simulink model "gbyk_rwd_tgtprob"  (R2015a)
settings: Solver=ode4  SolverMode=MultiTasking  StartTime=0.0  StopTime=inf  FixedStep=BKIN_STEP_TIME  RelTol=1e-3
StartFcn:
  |  warndlg('Dexterit-E models cannot run under simulation. Please compile your model and run it from within Dexterit-E.');set_param(bdroot,'SimulationCommand','stop')
model workspace (MAT data in the model file):
  BKIN_STEP_TIME = 0.00025
  col_x = 1
  col_y = 2
  INIT_COLOR = 5
  DELAY_POST_TRIAL = 8
  BKIN_KINEMATIC_FRAME_SIZE = 400
  HIT_COLOR = 6
  E_NO_EVENT = 0
  START_TARGET_COL = 1
  TARGET1_COL = 2
  TARGET2_COL = 3
  RWD_TARGET1_COL = 4
  RWD_TARGET2_COL = 5
  MAX_REACH_TIME_COL = 7
  K_DELAY_FIXED = 3
  K_DELAY_RAND = 4
  K_TRIGGER_VEL = 5
  K_TRIGGER_POS = 6
  K_THRESH_VELMAX = 7
  E_NEW_TRIAL = 1
  E_STAY_START = 2
  E_TARGET_TRIGGER = 5
  E_HIT_TARGET = 10
  E_MISS_TARGET = 11
  K_REWARD_VAL = 1
  VISUAL_RADIUS = 3
  LOGICAL_RADIUS = 4
  STROKE_WIDTH = 7
  TEXT_COLOR = 8
  LABEL_HEIGHT = 10
  E_TOO_SLOW = 20
  K_TONE_HIT_FREQUENCY = 8
  K_TONE_HIT_DURATION = 9
  K_TONE_ERROR_FREQUENCY = 12
  K_TONE_ERROR_DURATION = 13
  K_SCORETEXT_ROW = 2
  LABEL = 9
  E_TARGETS_ON = 3
  K_TONE_GO_FREQUENCY = 10
  K_TONE_GO_DURATION = 11
  DISPLAY_TRIAL_COL = 9
  E_SHOW_INSTRUCT = 25
  E_SHOW_SCORE = 26
  INSTRUCT_PAUSE_BTN = 2
  TARGET1_PROB_COL = 6
  TARGET_SIZE = 11
libraries: Video x6, slrtlib x5, General x3, KINARM_general x3, simulink x1, xpcnilib x1
CloseFcn:
  | rtwprivate ssgencode ModelCloseRequest b2lab2d
settings Model: ModifiedComment=chris -- Wed Feb 16 09:18:30 2005 -- Version 1.1384  ModifiedHistory=Feb 16/05 - Add error repeat, add offset ramp  ExtModeArmWhenConnect=off  ExtModeLogAll=off  Creator=Chris Grebeldinger  LastModifiedBy=User
settings SolverCC: EnableConcurrentExecution=on  AutoInsertRateTranBlk=on
settings DataIOCC: LimitDataPoints=off  SignalLoggingSaveFormat=ModelDataLogs  SaveOutput=off  SaveTime=off  SignalLoggingName=sigsOut
settings OptimizationCC: BlockReduction=off  BooleanDataType=off  OptimizeBlockIOStorage=off  BufferReuse=off  GlobalBufferReuse=off  ExpressionFolding=off  ExpressionDepthLimit=2147483647  LocalBlockOutputs=off  InitFltsAndDblsToZero=on
settings DebuggingCC: SaveWithParameterizedLinksMsg=none  UnderspecifiedInitializationDetection=Classic  MergeDetectMultiDrivingBlocksExec=none  SignalResolutionControl=TryResolveAllWithWarning  MultiTaskDSMMsg=warning  FcnCallInpInsideContextMsg=UseLocalSettings  StateNameClashWarn=warning  StrictBusMsg=ErrorOnBusTreatedAsVector
settings HardwareCC: ProdIntDivRoundTo=Zero  ProdEndianess=LittleEndian  ProdLongLongMode=on  ProdHWDeviceType=Generic->32-bit x86 compatible  TargetHWDeviceType=32-bit Generic
settings SFSimCC: SimCustomHeaderCode="#include \"stdlib.h\""  SFSimEcho=off  SimParseCustomCode=off
settings RTWCC: SystemTargetFile=slrt.tlc  TemplateMakefile=slrt_default_tmf  Description=Simulink Real-Time  CustomSourceCode="#include \"stdlib.h\""  RTWCompilerOptimization=on
settings CodeAppCC: MaxIdLength=63
settings SimulinkRealTimeCC: TargetFcnLib=ansi_tfl_tmw.mat  GeneratePreprocessorConditionals=Disable all  xPCisDownloadable=off  xPCisDefaultEnv=off

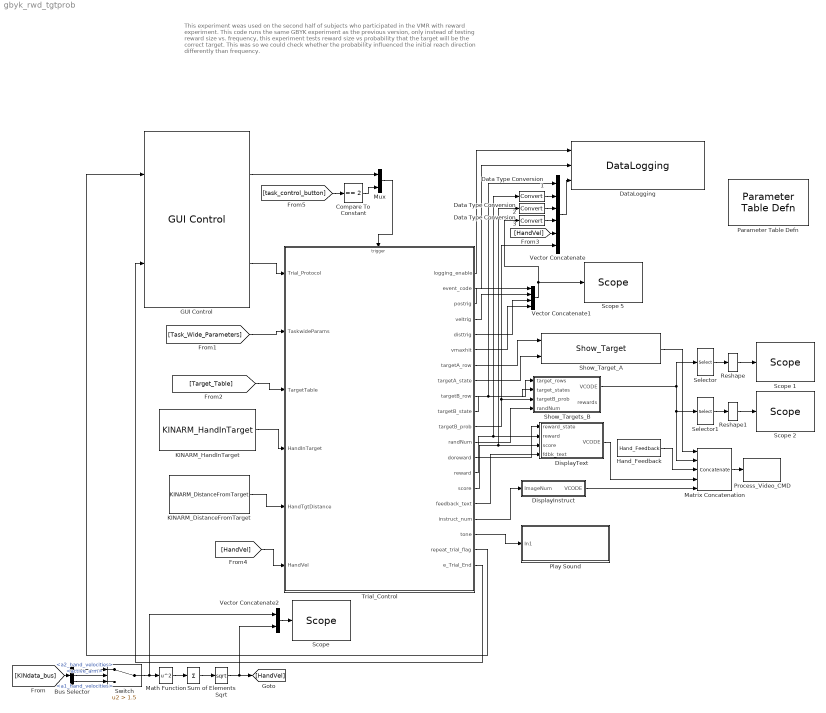
== system gbyk_rwd_tgtprob ==
  note: This experiment weas used on the second half of subjects who participated in the
      | VMR with reward experiment. This code runs the same GBYK experiment as the
      | previous version, only instead of testing reward size vs. frequency, this experiment
      | tests reward size vs probability that the target will be the correct target. This was
      | so we could check whether the probability influenced the initial reach direction
      | differently than frequency.
  Bus Selector : BusSelector  OutputSignals=Robot2.a2_hand_velocities,KINDataGeneral.active_arm,Robot1.a1_hand_velocities
  Compare To Constant : simulink/Logic and Bit Operations/Compare To Constant  relop===  const=2  OutDataTypeStr=boolean
  Data Type Conversion1 : DataTypeConversion
  Data Type Conversion2 : DataTypeConversion
  Data Type Conversion3 : DataTypeConversion
  DataLogging : General/DataLogging  log_event_codes=on  log_analog_inputs=on  show_time_remaining=off
      link override Poll KINARM/EPTorqueCMD: GotoTag=KINARMEPTorqueCMD
      link override Poll KINARM/TorqueCMD: GotoTag=KINARMTorqueCMD
  DisplayInstruct : Subsystem
  DisplayText : Subsystem
  GUI Control : General/GUI Control  target_type_str=Circle  Target_Type=1  XYcols=[1 2]  Vcols=3  Lcols=4  indices_padding=[0 0 0 0;0 0 0 0]  task_version=1.0  show_repeat_trial_flag=on  target_table_rows=32  load_table_rows=20  tp_table_rows=100
  Hand_Feedback : KINARM_general/Hand_Feedback  feedback_cntl_src=none
  KINARM_DistanceFromTarget : KINARM_general/KINARM_DistanceFromTarget  use_dominant_hand=on
  KINARM_HandInTarget : KINARM_general/KINARM_HandInTarget  use_dominant_hand=on  target_type=Circle  num_states=1  attribcol1=[LOGICAL_RADIUS]  attribcol2=[4]  attribcol3=[5]  attribcol4=[6]  attribcol5=[0]
  Math Function : Math  Operator=square  SaturateOnIntegerOverflow=on
  Matrix Concatenation : Concatenate  NumInputs=5  Mode=Multidimensional array
  Mux : Mux  Inputs=2
  Parameter Table Defn : General/Parameter Table Defn  ShowInLibBrowser=0
  Play Sound : Subsystem
  Process_Video_CMD : Video/Process_Video_CMD  video_delay=50
  Reshape : Reshape
  Reshape1 : Reshape
  "Scope " : slrtlib/Displays and Logging/Scope   scopeno=1  scopetype=Target  autostart=on  viewmode=Numerical  formatstr='%15.6f'  grid=on  ylimits=[0,0]  nosamples=250  noprepostsamples=0  interleave=1  triggermode=FreeRun  triggersignal=1  trigsignalfromport=off  triggerlevel=0.0  triggerslope=Either  triggerscope=1  triggersample=0  filename=data.dat  mode=Lazy  writesize=512  autorestart=off  dynamicfilemode=off  maxwritefilesize=512*1024^2
  Scope 1 : slrtlib/Displays and Logging/Scope   scopeno=2  scopetype=Target  autostart=on  viewmode=Numerical  formatstr='%15.6f'  grid=on  ylimits=[0,0]  nosamples=250  noprepostsamples=0  interleave=1  triggermode=FreeRun  triggersignal=1  trigsignalfromport=off  triggerlevel=0.0  triggerslope=Either  triggerscope=1  triggersample=0  filename=data.dat  mode=Lazy  writesize=512  autorestart=off  dynamicfilemode=off  maxwritefilesize=512*1024^2
  Scope 2 : slrtlib/Displays and Logging/Scope   scopeno=3  scopetype=Target  autostart=on  viewmode=Numerical  formatstr='%15.6f'  grid=on  ylimits=[0,0]  nosamples=250  noprepostsamples=0  interleave=1  triggermode=FreeRun  triggersignal=1  trigsignalfromport=off  triggerlevel=0.0  triggerslope=Either  triggerscope=1  triggersample=0  filename=data.dat  mode=Lazy  writesize=512  autorestart=off  dynamicfilemode=off  maxwritefilesize=512*1024^2
  Scope 5 : slrtlib/Displays and Logging/Scope   scopeno=6  scopetype=Target  autostart=on  viewmode=Numerical  formatstr='%15.6f'  grid=on  ylimits=[0,0]  nosamples=250  noprepostsamples=0  interleave=1  triggermode=FreeRun  triggersignal=1  trigsignalfromport=off  triggerlevel=0.0  triggerslope=Either  triggerscope=1  triggersample=0  filename=data.dat  mode=Lazy  writesize=512  autorestart=off  dynamicfilemode=off  maxwritefilesize=512*1024^2
  Selector : Selector  NumberOfDimensions=2  InputPortWidth=3  IndexOptions=Index vector (dialog),Index vector (dialog)  Indices=[1:2],[2 3 4 15 16]  OutputSizes=1,1
  Selector1 : Selector  NumberOfDimensions=2  InputPortWidth=3  IndexOptions=Index vector (dialog),Index vector (dialog)  Indices=[3:4],[2 3 4 9]  OutputSizes=1,1
  Show_Target_A : Video/Show_Target  target_type=Circle  num_states=2  attribcol1=[INIT_COLOR 0 0 VISUAL_RADIUS]  attribcol2=[HIT_COLOR 0 0 VISUAL_RADIUS]  attribcol3=[0 0 0 0]  attribcol4=[0 0 0 0]  attribcol5=[0 0 24 0]  stateindices_padding=[0 0 0 0 0 0 0;0 0 0 0 0 0 0;0 0 0 0 0 0 0;0 0 0 0 0 0 0;0 0 0 0 0 0 0]  source=dialog  opacity=100  target_display=Both subject and operator displays  num_col=4
  Show_Targets_B : Subsystem
  Sqrt : Sqrt  SaturateOnIntegerOverflow=on
  Sum of Elements : Sum  Inputs=+
  Switch : Switch  Criteria=u2 > Threshold  Threshold=1.5
  Trial_Control : Stateflow chart  TreatAsAtomicUnit=on
  Vector Concatenate : Concatenate  NumInputs=6
  Vector Concatenate1 : Concatenate  NumInputs=4
  Vector Concatenate2 : Concatenate
  wires:
  KINARM_HandInTarget/1 -> Trial_Control/4(HandInTarget)
  Show_Target_A/1 -> Matrix Concatenation/1
  GUI Control/2 -> Trial_Control/1(Trial_Protocol)
  Trial_Control/19(repeat_trial_flag) -> GUI Control/1
  Trial_Control/8(targetA_state) -> Show_Target_A/2
  Trial_Control/7(targetA_row) -> Show_Target_A/1
  Matrix Concatenation/1 -> Process_Video_CMD/1
  Hand_Feedback/1 -> Matrix Concatenation/3
  Show_Targets_B/1(VCODE) -> Selector/1, Selector1/1, Matrix Concatenation/2
  Trial_Control/9(targetB_row) -> Show_Targets_B/1(target_rows)
  Trial_Control/10(targetB_state) -> Vector Concatenate/1, Show_Targets_B/2(target_states)
  Trial_Control/1(logging_enable) -> DataLogging/1
  Trial_Control/2(event_code) -> DataLogging/2
  [KINdata_bus] -> Bus Selector/1
  KINARM_DistanceFromTarget/1 -> Trial_Control/5(HandTgtDistance)
  [Task_Wide_Parameters] -> Trial_Control/2(TaskwideParams)
  [Target_Table] -> Trial_Control/3(TargetTable)
  Trial_Control/13(doreward) -> DisplayText/1(reward_state)
  Trial_Control/20(e_Trial_End) -> GUI Control/2
  Trial_Control/14(reward) -> Data Type Conversion1/1, DisplayText/2(reward)
  Trial_Control/15(score) -> Data Type Conversion2/1, DisplayText/3(score)
  DisplayText/1(VCODE) -> Matrix Concatenation/4
  Vector Concatenate/1 -> DataLogging/3
  Data Type Conversion1/1 -> Vector Concatenate/2
  Data Type Conversion2/1 -> Vector Concatenate/3
  Trial_Control/16(feedback_text) -> DisplayText/4(fdbk_text)
  Selector/1 -> Reshape/1
  Reshape/1 -> Scope 1/1
  Trial_Control/3(postrig) -> Vector Concatenate1/1
  Trial_Control/4(veltrig) -> Vector Concatenate1/2
  Trial_Control/5(disttrig) -> Vector Concatenate1/3
  Trial_Control/6(vmaxhit) -> Vector Concatenate1/4
  Vector Concatenate1/1 -> Data Type Conversion3/1, Scope 5/1
  Data Type Conversion3/1 -> Vector Concatenate/4
  Vector Concatenate2/1 -> "Scope "/1
  Switch/1 -> Vector Concatenate2/1, Math Function/1
  Bus Selector/2 -> Switch/2  "<active_arm>"
  Bus Selector/3 -> Switch/3  "<a1_hand_velocities>"
  Bus Selector/1 -> Switch/1  "<a2_hand_velocities>"
  Math Function/1 -> Sum of Elements/1
  Sum of Elements/1 -> Sqrt/1
  [HandVel] -> Vector Concatenate/5
  [HandVel] -> Trial_Control/6(HandVel)
  Sqrt/1 -> Vector Concatenate2/2, [HandVel]
  Trial_Control/17(instruct_num) -> DisplayInstruct/1(ImageNum)
  DisplayInstruct/1(VCODE) -> Matrix Concatenation/5
  GUI Control/1 -> Mux/1
  [task_control_button] -> Compare To Constant/1
  Compare To Constant/1 -> Mux/2
  Mux/1 -> Trial_Control/Trigger
  Trial_Control/11(targetB_prob) -> Vector Concatenate/6, Show_Targets_B/3(targetB_prob)
  Selector1/1 -> Reshape1/1
  Reshape1/1 -> Scope 2/1
  Trial_Control/12(randNum) -> Show_Targets_B/4(randNum)
  Trial_Control/18(tone) -> Play Sound/1(In1)

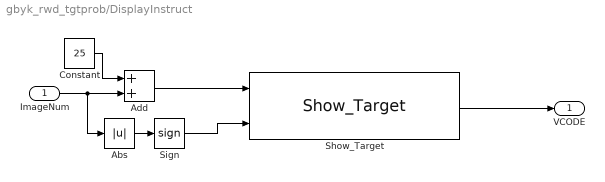
== system gbyk_rwd_tgtprob/DisplayInstruct ==
  ImageNum : Inport
  Abs : Abs
  Add : Sum
  Constant : Constant  Value=25
  Show_Target : Video/Show_Target  target_type=Rectangle  num_states=1  attribcol1=[INIT_COLOR 0 0 VISUAL_RADIUS LABEL_HEIGHT 0]  attribcol2=[6 6 0 3 0 0]  attribcol3=[0 0 0 0 0 0]  attribcol4=[0 0 0 0 0 0]  attribcol5=[0 0 24 0 0 0]  stateindices_padding=[0 0 0 0 0;0 0 0 0 0;0 0 0 0 0;0 0 0 0 0;0 0 0 0 0]  source=dialog  opacity=100  target_display=Both subject and operator displays  num_col=6
  Sign : Signum
  VCODE : Outport
  wires:
  ImageNum/1 -> Add/2, Abs/1
  Abs/1 -> Sign/1
  Show_Target/1 -> VCODE/1
  Add/1 -> Show_Target/1
  Constant/1 -> Add/1
  Sign/1 -> Show_Target/2

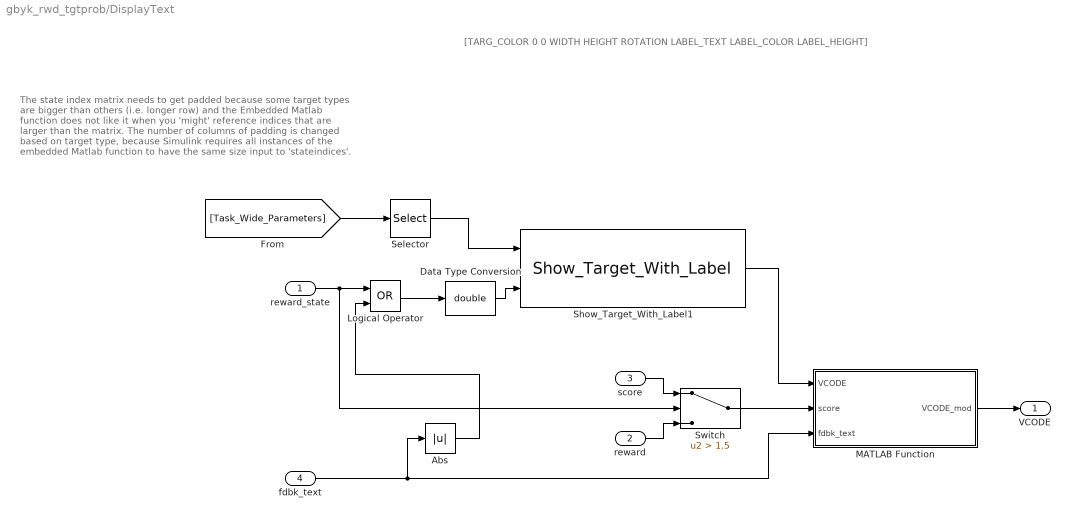
== system gbyk_rwd_tgtprob/DisplayText ==
  note: [TARG_COLOR 0 0 WIDTH HEIGHT ROTATION LABEL_TEXT LABEL_COLOR LABEL_HEIGHT]
  note: The state index matrix needs to get padded because
      | some target types are bigger than others (i.e. longer row)
      | and the Embedded Matlab function does not like it when you
      |  'might' reference indices that are larger than the matrix.
      |
      | The number of columns of padding is changed based on target
      | type, because Simulink requires all instances of the embedded
      | Matlab function to have the same size input to 'stateindices'.
  reward_state : Inport  OutDataTypeStr=double
  reward : Inport  Port=2  OutDataTypeStr=int32
  score : Inport  Port=3  OutDataTypeStr=int32
  fdbk_text : Inport  Port=4  OutDataTypeStr=int32
  Abs : Abs
  Data Type Conversion : DataTypeConversion  OutDataTypeStr=double
  Logical Operator : Logic  Operator=OR  AllPortsSameDT=off  OutDataTypeStr=boolean
  MATLAB Function : MATLAB Function  TreatAsAtomicUnit=on
  Selector : Selector  InputPortWidth=50  Indices=[K_SCORETEXT_ROW]
  Show_Target_With_Label1 : Video/Show_Target_With_Label  target_type=Rectangle  num_states=1  attribcol1=[INIT_COLOR 0 0 VISUAL_RADIUS VISUAL_RADIUS 0 LABEL TEXT_COLOR LABEL_HEIGHT]  attribcol2=[6 6 0 3 0 0 0 0 0]  attribcol3=[0 0 0 0 0 0 0 0 0]  attribcol4=[0 0 0 0 0 0 0 0 0]  attribcol5=[0 0 24 0 0 0 0 0 0]  stateindices_padding=[0 0;0 0;0 0;0 0;0 0]  source=dialog  opacity=100  target_display=Both subject and operator displays
  Switch : Switch  Criteria=u2 > Threshold  Threshold=1.5
  VCODE : Outport
  wires:
  reward_state/1 -> Logical Operator/1, Switch/2
  Show_Target_With_Label1/1 -> MATLAB Function/1(VCODE)
  MATLAB Function/1(VCODE_mod) -> VCODE/1
  score/1 -> Switch/1
  reward/1 -> Switch/3
  Switch/1 -> MATLAB Function/2(score)
  [Task_Wide_Parameters] -> Selector/1
  Selector/1 -> Show_Target_With_Label1/1
  Abs/1 -> Logical Operator/2
  Logical Operator/1 -> Data Type Conversion/1
  Data Type Conversion/1 -> Show_Target_With_Label1/2
  fdbk_text/1 -> MATLAB Function/3(fdbk_text), Abs/1

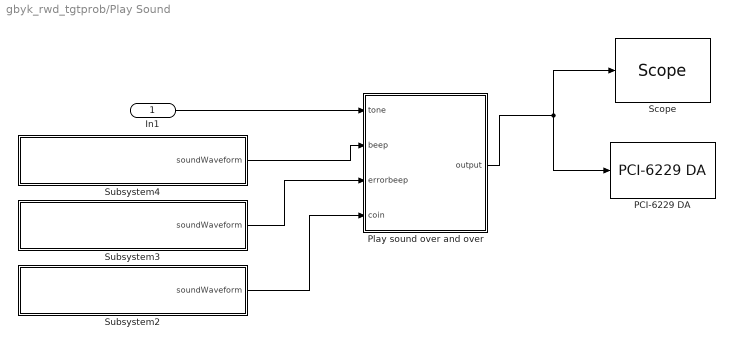
== system gbyk_rwd_tgtprob/Play Sound ==
  In1 : Inport
  PCI-6229 DA : xpcnilib/D//A/M Series/PCI-6229 DA  channel=[1]  reset=[1]  initValue=[0]  sampletime=-1  slot=-1
  Play sound over and over : MATLAB Function  TreatAsAtomicUnit=on
  "Scope " : slrtlib/Displays and Logging/Scope   scopeno=4  scopetype=Target  autostart=on  viewmode=Graphical redraw  formatstr='%15.6f'  grid=on  ylimits=[0,0]  nosamples=4000  noprepostsamples=0  interleave=1  triggermode=FreeRun  triggersignal=1  trigsignalfromport=off  triggerlevel=0.0  triggerslope=Either  triggerscope=1  triggersample=0  filename=data.dat  mode=Lazy  writesize=512  autorestart=off  dynamicfilemode=off  maxwritefilesize=512*1024^2
  Subsystem2 : Subsystem  mask(Load Waveform Into Variable){fileName=beep2}
      mask prompts: fileName "Name of .mat Data File (must be in current directory)"
      mask help: This block will load the .MAT file specified in the dialog, and put the first variable into a GoTo called 'soundWaveform'.
      mask init:
      | filenameFromMask = get_param(gcb, 'fileName');
      | 
      | try 
      | 	dataFromFile = load(filenameFromMask);
      | 	names = fieldnames(dataFromFile);
      | 	soundDataFromFile = dataFromFile.(names{1});
      | 	display(['Sound waveform from file ''' filenameFromMask ''' loaded.']);
      | catch ME
      | 	display(ME.message)
      | end
      mask Help:
      | Enter the name a .MAT file containing a single vector or matrix. The .MAT file must be located in the current directory.
      | 
      | The first variable from the .MAT file will be put into a Goto called 'soundWaveform'.
      mask Display: disp(['Load waveform from ''' filenameFromMask ''''])
  Subsystem3 : Subsystem  mask(Load Waveform Into Variable){fileName=beep1}
      mask prompts: fileName "Name of .mat Data File (must be in current directory)"
      mask help: This block will load the .MAT file specified in the dialog, and put the first variable into a GoTo called 'soundWaveform'.
      mask init: same as gbyk_rwd_tgtprob/Play Sound/Subsystem2
      mask Help:
      | Enter the name a .MAT file containing a single vector or matrix. The .MAT file must be located in the current directory.
      | 
      | The first variable from the .MAT file will be put into a Goto called 'soundWaveform'.
      mask Display: disp(['Load waveform from ''' filenameFromMask ''''])
  Subsystem4 : Subsystem  mask(Load Waveform Into Variable){fileName=beep}
      mask prompts: fileName "Name of .mat Data File (must be in current directory)"
      mask help: This block will load the .MAT file specified in the dialog, and put the first variable into a GoTo called 'soundWaveform'.
      mask init: same as gbyk_rwd_tgtprob/Play Sound/Subsystem2
      mask Help:
      | Enter the name a .MAT file containing a single vector or matrix. The .MAT file must be located in the current directory.
      | 
      | The first variable from the .MAT file will be put into a Goto called 'soundWaveform'.
      mask Display: disp(['Load waveform from ''' filenameFromMask ''''])
  wires:
  Play sound over and over/1(output) -> PCI-6229 DA/1, "Scope "/1
  Subsystem3/1(soundWaveform) -> Play sound over and over/3(errorbeep)
  Subsystem4/1(soundWaveform) -> Play sound over and over/2(beep)
  In1/1 -> Play sound over and over/1(tone)
  Subsystem2/1(soundWaveform) -> Play sound over and over/4(coin)

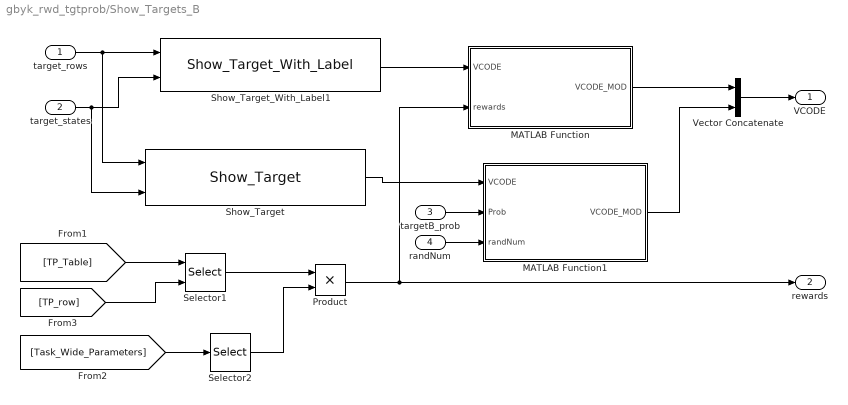
== system gbyk_rwd_tgtprob/Show_Targets_B ==
  target_rows : Inport
  target_states : Inport  Port=2
  targetB_prob : Inport  Port=3
  randNum : Inport  Port=4
  MATLAB Function : MATLAB Function  TreatAsAtomicUnit=on
  MATLAB Function1 : MATLAB Function  TreatAsAtomicUnit=on
  Product : Product
  Selector1 : Selector  NumberOfDimensions=2  InputPortWidth=100  IndexOptions=Index vector (port),Index vector (dialog)  Indices=[],[RWD_TARGET1_COL RWD_TARGET2_COL]  OutputSizes=1,1
  Selector2 : Selector  InputPortWidth=50  Indices=[K_REWARD_VAL]
  Show_Target : Video/Show_Target  target_type=Rectangle  num_states=3  attribcol1=[INIT_COLOR INIT_COLOR STROKE_WIDTH TARGET_SIZE TARGET_SIZE 0]  attribcol2=[INIT_COLOR INIT_COLOR STROKE_WIDTH TARGET_SIZE TARGET_SIZE 0]  attribcol3=[HIT_COLOR HIT_COLOR STROKE_WIDTH TARGET_SIZE TARGET_SIZE 0]  attribcol4=[0 0 0 0 0 0]  attribcol5=[0 0 24 0 0 0]  stateindices_padding=[0 0 0 0 0;0 0 0 0 0;0 0 0 0 0;0 0 0 0 0;0 0 0 0 0]  source=dialog  opacity=100  target_display=Both subject and operator displays  num_col=6
  Show_Target_With_Label1 : Video/Show_Target_With_Label  target_type=Circle  num_states=3  attribcol1=[0 0 0 VISUAL_RADIUS LABEL TEXT_COLOR LABEL_HEIGHT]  attribcol2=[0 0 0 VISUAL_RADIUS LABEL TEXT_COLOR LABEL_HEIGHT]  attribcol3=[0 0 0 VISUAL_RADIUS LABEL TEXT_COLOR LABEL_HEIGHT]  attribcol4=[0 0 0 0 0 0 0]  attribcol5=[0 0 24 0 0 0 0]  stateindices_padding=[0 0 0 0;0 0 0 0;0 0 0 0;0 0 0 0;0 0 0 0]  source=dialog  opacity=100  target_display=Both subject and operator displays
  Vector Concatenate : Concatenate  Mode=Multidimensional array
  VCODE : Outport
  rewards : Outport  Port=2
  wires:
  [TP_Table] -> Selector1/1
  Selector1/1 -> Product/1
  [Task_Wide_Parameters] -> Selector2/1
  Selector2/1 -> Product/2
  [TP_row] -> Selector1/2
  target_rows/1 -> Show_Target/1, Show_Target_With_Label1/1
  target_states/1 -> Show_Target/2, Show_Target_With_Label1/2
  Show_Target_With_Label1/1 -> MATLAB Function/1(VCODE)
  Product/1 -> MATLAB Function/2(rewards), rewards/1
  Show_Target/1 -> MATLAB Function1/1(VCODE)
  targetB_prob/1 -> MATLAB Function1/2(Prob)
  Vector Concatenate/1 -> VCODE/1
  MATLAB Function/1(VCODE_MOD) -> Vector Concatenate/1
  MATLAB Function1/1(VCODE_MOD) -> Vector Concatenate/2
  randNum/1 -> MATLAB Function1/3(randNum)

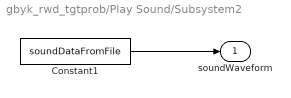
== system gbyk_rwd_tgtprob/Play Sound/Subsystem2 ==
  Constant1 : Constant  Value=soundDataFromFile
  soundWaveform : Outport
  wires:
  Constant1/1 -> soundWaveform/1

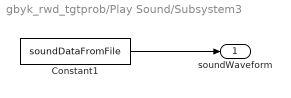
== system gbyk_rwd_tgtprob/Play Sound/Subsystem3 ==
  Constant1 : Constant  Value=soundDataFromFile
  soundWaveform : Outport
  wires:
  Constant1/1 -> soundWaveform/1

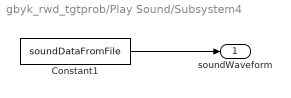
== system gbyk_rwd_tgtprob/Play Sound/Subsystem4 ==
  Constant1 : Constant  Value=soundDataFromFile
  soundWaveform : Outport
  wires:
  Constant1/1 -> soundWaveform/1

== stateflow chart gbyk_rwd_tgtprob/Trial_Control ==
  settings: sampleTime=0.001
  state MainTrial
    state ShowStartTarget/
      // Turn on first target, enable data logging, and wait for a specified time or until the hand is in the target.
      targetA_row = Trial_Protocol[START_TARGET_COL];
      targetA_state = 1;
      logging_enable = 1;
      veltrig = 0;
      postrig = 0;
      disttrig = 0;
      vmaxhit = 0;
      targetB_state[1] = 0;
      targetB_state[2] = 0;
      tone = 0;
    state StayAtFirstTarget/
      // Log an event that target was reached and wait for a specified time.
      // The wait time may have both a fixed and a random component. The hand must stay in the target for the full wait time.
      event_code = E_STAY_START;
      //targetA_state = 1;
      tickCount = TaskwideParams[K_DELAY_FIXED] + TaskwideParams[K_DELAY_RAND] * rand() / RAND_MAX;
      //Show targets before the go tone - allows for comparison
      targetB_row[1] = Trial_Protocol[TARGET1_COL];
      targetB_row[2] = max(Trial_Protocol[TARGET2_COL],1);
      targetB_state[1] = 1;
      targetB_state[2] = double(Trial_Protocol[TARGET2_COL] > 0);
      targetB_prob[1] = Trial_Protocol[TARGET1_PROB_COL];
      targetB_prob[2] = 1-Trial_Protocol[TARGET1_PROB_COL];
      //This random number is used to pick a png file for the target
      randNum[1] = floor(rand()/RAND_MAX*(50/5));
      randNum[2] = floor(rand()/RAND_MAX*(50/5));
    state ShowReachTargets/
      // Turn on all reach targets and log an event indicating this has occurred. Then wait until the hand is the target or until a specified time has elapsed.
      event_code = E_TARGETS_ON;
      tickCount = Trial_Protocol[MAX_REACH_TIME_COL];
      tone = 1;
      during:
      //handvel2d = sqrt((HandVel[1])^2 + (HandVel[2])^2);
      veltrig =  (HandVel > TaskwideParams[K_TRIGGER_VEL]);
      postrig = abs(HandTgtDistance[targetA_row]) > TaskwideParams[K_TRIGGER_POS];
    state TriggerTarget/
      //shut off second reach target
      event_code = E_TARGET_TRIGGER;
      targetB_state[1] = 2;
      targetB_state[2] = 0;
      during:
      postrig = HandInTarget[targetB_row[1]]==1;
      disttrig = abs(HandTgtDistance[targetA_row]) > (abs(TargetTable[targetB_row[1]][col_y] - TargetTable[targetA_row][col_y]) + TargetTable[targetB_row[1]][VISUAL_RADIUS])*0.01;
      vmaxhit = (vmaxhit || (HandVel > TaskwideParams[K_THRESH_VELMAX]));  //(sqrt(HandVel[1]^2 + HandVel[2]^2)
    state HitTarget/
      // Log a successful hit
      event_code = E_HIT_TARGET;
      targetB_state[1] = 3;
      doreward = double((Trial_Protocol[RWD_TARGET1_COL] > 0) || (Trial_Protocol[RWD_TARGET2_COL] > 0));
      reward = Trial_Protocol[RWD_TARGET1_COL]*TaskwideParams[K_REWARD_VAL];
      score += reward;
      tone = 3;
      tickCount = 500;
    state MissTarget/
      // Log a target miss
      event_code = E_MISS_TARGET;
      targetB_state[1] = 0;
      reward = 0;
      doreward = 0;
      tickCount = 500;
    state TooSlow/
      // Log a bad trial
      event_code = E_TOO_SLOW;
      targetB_state[1] = 0;
      repeat_trial_flag = 1;
      reward = 0;
      doreward = 0;
      //feedback_text = -1;
      tone = 2
      tickCount = 500;
    state EndOfTrial/
      // Set the post-trial delay.
      tickCount = Trial_Protocol[DELAY_POST_TRIAL];
    ShowStartTarget -> StayAtFirstTarget : [HandInTarget[targetA_row] == 1]
    StayAtFirstTarget -> ShowStartTarget [order 2] : [HandInTarget[targetA_row] == 0]
    StayAtFirstTarget -> ShowReachTargets [order 1] : after(tickCount, e_clk)
    ShowReachTargets -> TooSlow [order 1] : after(tickCount, e_clk)/
        | feedback_text = -2;
        | //if the trial times out it is an error
    ShowReachTargets -> TriggerTarget [order 2] : [after(1,e_clk) && (veltrig || postrig)]
        | //when the hand velocity pr position exceeds the threshold
        | //shut off the second target
    TriggerTarget -> HitTarget [order 3] : [after(1,e_clk) && postrig && vmaxhit]
        | //check if hit the target and moved fast enough
    TriggerTarget -> MissTarget [order 2] : [after(1,e_clk) && (disttrig && !postrig) && vmaxhit]/
        | //check if missed the target but moved fast enough
    TriggerTarget -> TooSlow [order 1] : [(after(1,e_clk) && (disttrig || postrig) && vmaxhit == 0) || after(tickCount, e_clk)]/
        | feedback_text = -1;
        | //check if missed the target but moved fast enough
    MissTarget -> EndOfTrial : after(tickCount, e_clk)
    HitTarget -> EndOfTrial : after(tickCount, e_clk)
    TooSlow -> EndOfTrial : after(tickCount, e_clk)
  state Initialize/
    // Both the targets and data logging are initially off.
    targetA_state = 0;
    targetB_state[1] = 0;
    targetB_state[2] = 0;
    logging_enable = 0;
    score = 0;
    reward = 0;
    doreward = 0;
    feedback_text = 0;
    repeat_trial_flag = 0;
  state EndInstructPause/
    instruct_num = 0;
    tickCount = Trial_Protocol[DELAY_POST_TRIAL];
    logging_enable = 1;
    score = 0;
  state Ending/
    //end the special "show score" state
    //score = 0;
    e_Trial_End;
  state ReturnToStart1/
    targetA_state=1;
    targetB_state[1] = 0;
    targetB_state[2] = 0;
    feedback_text = 0;
    doreward = 0;
    repeat_trial_flag = 0;
    logging_enable = 1;
  state InstructWaitState/
    //"pause" here until the button has been clicked
  state ShowScoreState/
    event_code = E_SHOW_SCORE;
    targetA_state = 0;
    targetB_state[1] = 0;
    targetB_state[2] = 0;
    doreward = 2;
    tickCount = Trial_Protocol[MAX_REACH_TIME_COL];
    logging_enable = 0;
  state ShowInstructState/
    event_code = E_SHOW_INSTRUCT;
    targetA_state = 0;
    targetB_state[1] = 0;
    targetB_state[2] = 0;
    doreward = 0;
    instruct_num = Trial_Protocol[DISPLAY_TRIAL_COL];
    tickCount = Trial_Protocol[MAX_REACH_TIME_COL];
    logging_enable = 0;
  state Inter_Trial_State/
    // Turn off both targets, turn off data logging, reset the
    // event code, and send the e_Trial_End Stateflow event.
    event_code = 0;
    targetA_state = 1;
    targetB_state[1] = 0;
    targetB_state[2] = 0;
    feedback_text = 0;
    doreward = 0;
    e_Trial_End;
  (default) -> Initialize
  Initialize -> ShowStartTarget [order 1] : [Trial_Protocol[DISPLAY_TRIAL_COL] == 0]
  ReturnToStart1 -> ShowStartTarget : after(1, e_clk)/
  Initialize -> ShowInstructState [order 2] : [Trial_Protocol[DISPLAY_TRIAL_COL] > 0]
      | //in case we start with an instruction trial
  Ending -> (junction 91) : after(1,e_clk)
  (junction 91) -> EndInstructPause [order 1] : [Trial_Protocol[DISPLAY_TRIAL_COL] == 0]/
      | //continue if a regular trial comes after!
  (junction 91) -> ShowInstructState [order 2] : //so we can show the score and then show instructions
      | [Trial_Protocol[DISPLAY_TRIAL_COL] > 0]
  InstructWaitState -> Ending : e_cntl_btn/
      | event_code = 22;
  EndInstructPause -> ReturnToStart1 : after(tickCount,e_clk)
  ShowScoreState -> Ending : after(tickCount,e_clk)
  ShowInstructState -> InstructWaitState : after(tickCount,e_clk)
  (junction 86) -> ReturnToStart1 [order 3] : [Trial_Protocol[DISPLAY_TRIAL_COL] == 0]
  (junction 86) -> ShowScoreState [order 1] : [Trial_Protocol[DISPLAY_TRIAL_COL] == -1]
  (junction 86) -> ShowInstructState [order 2] : [Trial_Protocol[DISPLAY_TRIAL_COL] > 0]
  Inter_Trial_State -> (junction 86) : after(1,e_clk)
  MainTrial -> Inter_Trial_State : e_ExitTrialNow/
      | tickCount = 1;
  EndOfTrial -> Inter_Trial_State : after(tickCount,e_clk)
  data: logging_enable output boolean; Trial_Protocol input double; TaskwideParams input double; TargetTable input double; HandInTarget input double; event_code output uint16 [0..] =0; postrig output boolean; veltrig output boolean; disttrig output boolean; vmaxhit output boolean; targetA_row output [1..32]; targetA_state output double; targetB_row output double size=[2]; targetB_state output double size=[2]; targetB_prob output double size=[2]; randNum output double size=2; tickCount local double; RAND_MAX constant double =32767; HandTgtDistance input double; HandVel input double; doreward output double; reward output int32; score output int32; feedback_text output int32; instruct_num output double; tone output double; repeat_trial_flag output double
  data targetA_row settings: description=index of the row currently being used in the TargetTable
  events: e_clk input RISING_EDGE_EVENT; e_ExitTrialNow input EITHER_EDGE_EVENT; e_Trial_End output EITHER_EDGE_EVENT; e_cntl_btn input EITHER_EDGE_EVENT

== matlab function gbyk_rwd_tgtprob/Show_Targets_B/MATLAB Function ==
  data: VCODE input; VCODE_MOD output; rewards input
function VCODE_MOD  = rwd_tgt(VCODE,rewards)
%#codegen

%write out the reward value for each target

VCODE_MOD = VCODE;

%rewards = rwd_multipliers*rwd_val;

VCODE_MOD(:,4) = VCODE_MOD(:,4)+2*VCODE_MOD(:,10); %shift the label vertically above the target

for a = 1:length(rewards)

    if any(rewards)>0
        jj = 1;
        label = rewards(a);
        
        if (label < 10)
            VCODE_MOD(a, jj + 14) = int32(label+int32('0'));
            
        elseif (label < 100) %score < $1
            n1 = int32(floor(double(label)/10));  %we need to cast score to a double otherwise the arithmetic is wrong!
            n2 = label - n1*10;
        
            VCODE_MOD(a, jj + 14) = int32(n1+int32('0'));
            jj = jj+1;
            VCODE_MOD(a, jj + 14) = int32(n2+int32('0'));
        else %label < 1000
            n1 = int32(floor(double(label)/100));  %we need to cast score to a double otherwise the arithmetic is wrong!
            n2 = label - n1*100;
            n2 = int32(floor(double(n2)/100));  %we need to cast score to a double otherwise the arithmetic is wrong!
            n3 = label - n1*100 - n2*10;
        
            VCODE_MOD(a, jj + 14) = int32(n1+int32('0'));
            jj = jj+1;
            VCODE_MOD(a, jj + 14) = int32(n2+int32('0'));
            jj = jj+1;
            VCODE_MOD(a, jj + 14) = int32(n3+int32('0'));
        end
        VCODE_MOD(a,jj + 1 + 14) = 0; %terminate string
    else
        VCODE_MOD(a,15) = 0; %terminate string
    end
end

== matlab function gbyk_rwd_tgtprob/Show_Targets_B/MATLAB Function1 ==
  data: VCODE input; VCODE_MOD output; Prob input; randNum input
function VCODE_MOD  = rwd_tgt(VCODE,Prob,randNum)
%#codegen

%change the target color to reflect its probability

VCODE_MOD = VCODE;
imgnum = [0,0];
if randNum(1) == randNum(2)
    randNum(2) = randNum(2) + 1; %add one to randNum(2) if randNums equivalent
    if randNum(2) > 9 
        randNum(2) = 1; %arbitry int 1:10 as a default if randNum = [9,9]
    end
end

for a = 1:size(VCODE_MOD,1)
    
    imgnum(a) = -3+28.6667*Prob(a)-50*Prob(a) ^2+33.3333*Prob(a)^3;
    imgnum(a) = floor((50/5)* imgnum(a) - randNum(a));
    VCODE_MOD(a, 5) = -imgnum(a);
    
    
    
    %we assume the target color coming in is when P = 1, and that when P =
    %0 the color is 0. Instead of modifying the color, we can just change
    %its transparency by modulating VCODE(9).
    
    %rescale the probability, since 10% is too dim and not visible...
    %prob = Prob(a)/2+0.4; %rescale and recenter
    %prob = (Prob(a)-0.5)/2 + 0.5; %simple range rescale
    %     prob = (Prob(a)-0.5)*1.3+0.5+0.1; %range rescale and linear shift
    %     if prob > 1
    %         prob = 1;
    %     elseif prob < 0
    %         prob = 0;
    %     end
    %
    %     % Set the opacity value, on a range from 100 to 0.
    % 	VCODE_MOD(a, 9) = round(prob*100);
    
    % change tgt from red to blue based on probability (low probability is red)
    
    %prob = -1 + 7.16666*Prob(a) - 12.5*Prob(a)^2 + 8.33333*Prob(a)^3; %transforms [.2 .3 .5 .7 .8] into [0 .25 .5 .75 1]
    %prob = -0.6 + 3.86667*Prob(a) - 5*Prob(a)^2 + 3.33333*Prob(a)^3; %transforms [.2 .3 .5 .7 .8] into [0 .2 .5 .8 1]
    %prob = -1.4 + 10.4667*Prob(a) - 20*Prob(a)^2 + 13.3333*Prob(a)^3; %transforms [.2 .3 .5 .7 .8] into [0 .3 .5 .7 1]
    %prob = -0.7 + 5.73333*Prob(a) - 10*Prob(a)^2 + 6.66667*Prob(a)^3; %transforms [.2 .3 .5 .7 .8] into [.1 .3 .5 .7 .9]
    %prob = -0.35 + 3.36667*Prob(a) - 5*Prob(a)^2 + 3.33333*Prob(a)^3; %transforms [.2 .3 .5 .7 .8] into [.15 .3 .5 .7 .85]
    %prob = -0.75 + 6.66667*Prob(a) - 12.5*Prob(a)^2 + 8.33333*Prob(a)^3; %transforms [.2 .3 .5 .7 .8] into [.15 .35 .5 .65 .85]
    %prob = -0.4 + 4.3*Prob(a) - 7.5*Prob(a)^2 + 5*Prob(a)^3; %transforms [.2 .3 .5 .7 .8] into [.2 .35 .5 .65 .8]
    %prob = -0.45 + 5.23333 *Prob(a) - 10*Prob(a)^2 + 6.66667*Prob(a)^3;  %transforms [.2 .3 .5 .7 .8] into [.25 .4 .5 .6 .8]
    
%     if prob > 1
%         prob = 1;
%     elseif prob < 0
%         prob = 0;
%     end
%     
%         RRRGGGBBB = 1000000*(255-round(prob*255))+(round(prob*255));
%         blue = cast(mod(RRRGGGBBB, 1000), 'uint32');
%         green = cast(mod(RRRGGGBBB - blue, 1000000) / 1000, 'uint32');
%         red = cast((RRRGGGBBB - (green * 1000) - blue) / 1000000, 'uint32');
%         
%         RRGGBBAA = bitshift(red, 16) + bitshift(green, 8) + blue;
%         
%         VCODE_MOD(a, [5,6]) = RRGGBBAA;


end

== matlab function gbyk_rwd_tgtprob/Play Sound/Play sound over and over ==
  data: tone input; output output; beep input; errorbeep input; coin input
function output = fcn(tone,beep,errorbeep,coin)
%#codegen

persistent t last_tone_state
if isempty(t), t = 0; end
if isempty(last_tone_state), last_tone_state = 0; end

trigger = last_tone_state ~= tone;
if trigger > 0
    last_tone_state = tone;
end

output = 0;		% default
if t == 0 && trigger > 0
	% start the playing of the sound.
	t = t + 1;
end

if tone == 1
    data = beep;
elseif tone == 2
    data = errorbeep;
elseif tone == 3
    data = coin;
else 
    t = 0;
    data = 0;
end

if t > 0
	output = data(t);
	if t == length(data)
		t = 0;
	else
		t = t + 1;
	end
end

== matlab function gbyk_rwd_tgtprob/DisplayText/MATLAB Function ==
  data: VCODE input; score input; VCODE_mod output; fdbk_text input
function VCODE_mod = fcn(VCODE,score,fdbk_text)


VCODE_mod = VCODE;

if (fdbk_text == 0)  %if this is zero, show the score
       
    
    %score is in cents. potentially need to convert to dollars
    
    if (score < 10)
        text1 = 'You earned ';
        text2 = ' cents!';
        
        textout = [text1 int2char(int32(score)) text2];
        
    elseif (score < 100) %score < $1
        text1 = 'You earned ';
        text2 = ' cents!';
        
        n1 = int32(floor(double(score)/10));  %we need to cast score to a double otherwise the arithmetic is wrong!
        n2 = score - n1*10;
        
        textout = [text1 int2char(int32(n1)) int2char(int32(n2)) text2];
        
    else %score > $1, convert to dollars to keep the score readable
        text1 = 'You earned $';
        text2 = '.';
        text3 = '!';
        
        dollars = int32(floor(double(score)/100));
        if (dollars >= 10) %double digit dollar value
            n1d = int32(floor(double(dollars)/10));
            n2d = dollars - n1d*10;
            textdollars = [int2char(int32(n1d)) int2char(int32(n2d))];
        else %single digit
            textdollars = int2char(int32(dollars));
        end
        
        cents = score-dollars*100;
        if (cents < 10)
            textcents = ['0' int2char(int32(cents))];
        else
            n1 = int32(floor(double(cents)/10));
            n2 = round(cents - n1*10);
            textcents = [int2char(int32(n1)) int2char(int32(n2))];
        end
        
        textout = [text1 textdollars text2 textcents text3];
        
    end
    
elseif (fdbk_text == 1) 
    %print "too fast"
    textout = 'Too Fast!';
    
    
elseif (fdbk_text == 2) 
    %print "too fast"
    textout = 'Too Early!';

elseif (fdbk_text == -1) 
    %print "too slow"
    
    textout = 'Too Slow!';

elseif (fdbk_text == -2) 
    %print "too fast"
    textout = 'Too Late!';


else
    textout = '';
    
end
    

%the first character is VCODE(15)
%need to translate text into ascii:
textnum = double(textout); %this quickly casts each char into a number

%make sure we won't overflow the VCODE: no more than 50 chars! we will
%clip off anything that overflows.
VCODE_mod(1,15:min([15+length(textout),64])) = textnum(1:min([length(textnum),50])); %write out as many the characters as possible into the VCODE
VCODE_mod(1,min([15+length(textout)+1,64])) = 0;  %terminate the string!



function s = int2char(n)

n = mod(n,10); %make sure we only have 1 digit or we will get a weird character!

s = char(n+int32('0')); %// add the character
